simulink model "Platoon_Local_new_2015a"  (R2015a)
settings: Solver=ode45  StartTime=0.0  StopTime=100  RelTol=1e-3
undefined symbols (not defined in the file or in its folder): L, point_character, theta0, V0, x0, z0
undefined symbols (not defined in the file): theta1, theta2, theta3, theta4, x1, x2, x3, x4, z1, z2, z3, z4
settings Model: Creator=Prajval  LastModifiedBy=Aman
settings DataIOCC: LimitDataPoints=off  SaveFormat=Dataset
settings HardwareCC: ProdBitPerPointer=64  ProdLargestAtomicFloat=Float  ProdIntDivRoundTo=Zero  ProdEndianess=LittleEndian  ProdHWDeviceType=Specified
settings ModelReferenceCC: PropagateSignalLabelsOutOfModel=on

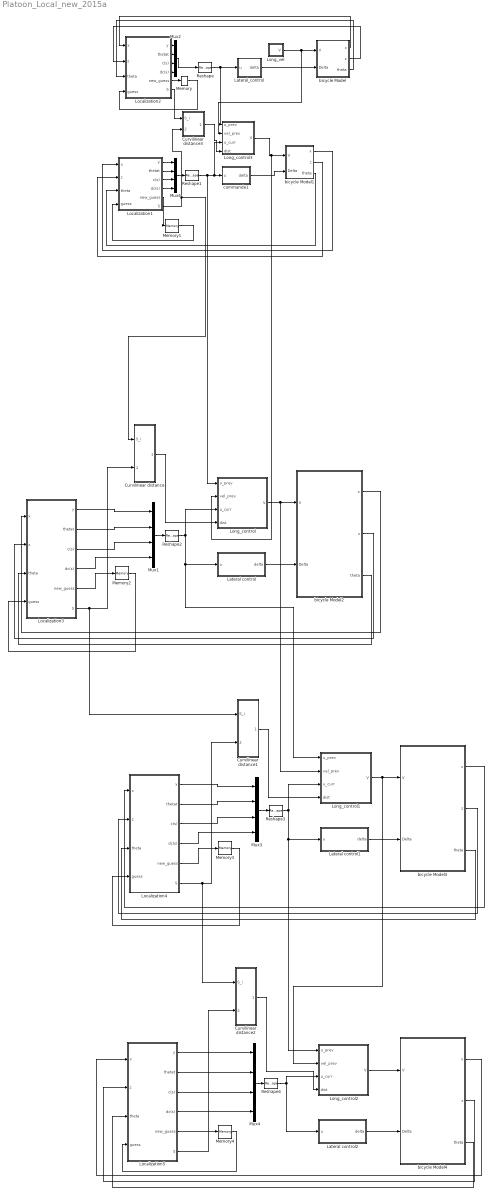
== system Platoon_Local_new_2015a ==
  Curvilinear distance : Subsystem
  Curvilinear distance1 : Subsystem
  Curvilinear distance2 : Subsystem
  Curvilinear distance3 : Subsystem
  Lateral control : MATLAB Function  TreatAsAtomicUnit=on
      settings: PermitHierarchicalResolution=ParametersOnly
  Lateral control1 : MATLAB Function  TreatAsAtomicUnit=on
      settings: PermitHierarchicalResolution=ParametersOnly
  Lateral control2 : MATLAB Function  TreatAsAtomicUnit=on
      settings: PermitHierarchicalResolution=ParametersOnly
  Lateral_control : MATLAB Function  TreatAsAtomicUnit=on
      settings: PermitHierarchicalResolution=ParametersOnly
  Localization1 : Subsystem
  Localization2 : Subsystem
  Localization3 : Subsystem
  Localization4 : Subsystem
  Localization5 : Subsystem
  Long_control : Subsystem
  Long_control1 : Subsystem
  Long_control2 : Subsystem
  Long_control3 : Subsystem
  Long_vel : Subsystem
  Memory{,1..4} (5 alike) : Memory  X0=1
  Mux{1..4,6} (5 alike) : Mux
  Reshape{,1..4} (5 alike) : Reshape  OutputDimensionality=Customize  OutputDimensions=[1,4]
  bicycle Model : Subsystem  mask{L=L, x0=x0, z0=z0, theta0=theta0}
      mask prompts: L "Wheelbase"
  bicycle Model1 : Subsystem  mask{L=L, x0=x1, z0=z1, theta0=theta1}
      mask prompts: L "Wheelbase"
  bicycle Model2 : Subsystem  mask{L=L, x0=x2, z0=z2, theta0=theta2}
      mask prompts: L "Wheelbase"
  bicycle Model3 : Subsystem  mask{L=L, x0=x3, z0=z3, theta0=theta3}
      mask prompts: L "Wheelbase"
  bicycle Model4 : Subsystem  mask{L=L, x0=x4, z0=z4, theta0=theta4}
      mask prompts: L "Wheelbase"
  commande1 : MATLAB Function  TreatAsAtomicUnit=on
      settings: PermitHierarchicalResolution=ParametersOnly
  wires:
  Lateral_control/1(delta) -> bicycle Model/2("Delta ")
  commande1/1(delta) -> bicycle Model1/2("Delta ")
  Mux6/1 -> Reshape1/1
  Localization2/3(c(s)) -> Mux2/3
  Localization2/2(thetat) -> Mux2/2
  Localization2/1(y) -> Mux2/1
  Reshape/1 -> Long_control3/1(u_prev), Lateral_control/1(u)
  Localization2/4(dc(s)) -> Mux2/4
  Mux2/1 -> Reshape/1
  Localization2/5("new_guess ") -> Memory/1
  bicycle Model/1(x) -> Localization2/1(x)
  bicycle Model/2(z) -> Localization2/2(z)
  bicycle Model/3(theta) -> Localization2/3(theta)
  Memory/1 -> Localization2/4(guess)
  Localization1/1(y) -> Mux6/1
  Localization1/2(thetat) -> Mux6/2
  Localization1/3(c(s)) -> Mux6/3
  Localization1/4(dc(s)) -> Mux6/4
  Localization1/5("new_guess ") -> Memory1/1
  Memory1/1 -> Localization1/4(guess)
  Localization1/6(S) -> Curvilinear distance3/2(S_i+1), Curvilinear distance/1(S_i)
  Reshape1/1 -> commande1/1(u), Long_control3/3(u_curr), Long_control/1(u_prev)
  bicycle Model1/1(x) -> Localization1/1(x)
  bicycle Model1/2(z) -> Localization1/2(z)
  bicycle Model1/3(theta) -> Localization1/3(theta)
  Lateral control/1(delta) -> bicycle Model2/2("Delta ")
  Mux1/1 -> Reshape2/1
  Localization3/1(y) -> Mux1/1
  Localization3/2(thetat) -> Mux1/2
  Localization3/3(c(s)) -> Mux1/3
  Localization3/4(dc(s)) -> Mux1/4
  Localization3/5("new_guess ") -> Memory2/1
  Reshape2/1 -> Long_control1/1(u_prev), Lateral control/1(u), Long_control/3(u_curr)
  bicycle Model2/1(x) -> Localization3/1(x)
  bicycle Model2/2(z) -> Localization3/2(z)
  bicycle Model2/3(theta) -> Localization3/3(theta)
  Long_control/1(V) -> Long_control1/2(vel_prev), bicycle Model2/1(V)
  Memory2/1 -> Localization3/4(guess)
  Localization3/6(S) -> Curvilinear distance1/1(S_i), Curvilinear distance/2(S_i+1)
  Curvilinear distance/1(dist) -> Long_control/4(dist)
  Lateral control1/1(delta) -> bicycle Model3/2("Delta ")
  Mux3/1 -> Reshape3/1
  Localization4/1(y) -> Mux3/1
  Localization4/2(thetat) -> Mux3/2
  Localization4/3(c(s)) -> Mux3/3
  Localization4/4(dc(s)) -> Mux3/4
  Localization4/5("new_guess ") -> Memory3/1
  Reshape3/1 -> Long_control2/1(u_prev), Lateral control1/1(u), Long_control1/3(u_curr)
  bicycle Model3/1(x) -> Localization4/1(x)
  bicycle Model3/2(z) -> Localization4/2(z)
  bicycle Model3/3(theta) -> Localization4/3(theta)
  Long_control1/1(V) -> Long_control2/2(vel_prev), bicycle Model3/1(V)
  Memory3/1 -> Localization4/4(guess)
  Curvilinear distance1/1(dist) -> Long_control1/4(dist)
  Lateral control2/1(delta) -> bicycle Model4/2("Delta ")
  Mux4/1 -> Reshape4/1
  Localization5/1(y) -> Mux4/1
  Localization5/2(thetat) -> Mux4/2
  Localization5/3(c(s)) -> Mux4/3
  Localization5/4(dc(s)) -> Mux4/4
  Localization5/5("new_guess ") -> Memory4/1
  Reshape4/1 -> Long_control2/3(u_curr), Lateral control2/1(u)
  bicycle Model4/1(x) -> Localization5/1(x)
  bicycle Model4/2(z) -> Localization5/2(z)
  bicycle Model4/3(theta) -> Localization5/3(theta)
  Long_control2/1(V) -> bicycle Model4/1(V)
  Memory4/1 -> Localization5/4(guess)
  Localization5/6(S) -> Curvilinear distance2/2(S_i+1)
  Curvilinear distance2/1(dist) -> Long_control2/4(dist)
  Localization4/6(S) -> Curvilinear distance2/1(S_i), Curvilinear distance1/2(S_i+1)
  Long_vel/1(V) -> Long_control3/2(vel_prev), bicycle Model/1(V)
  Localization2/6(S) -> Curvilinear distance3/1(S_i)
  Long_control3/1(V) -> Long_control/2(vel_prev), bicycle Model1/1(V)
  Curvilinear distance3/1(dist) -> Long_control3/4(dist)

== system Platoon_Local_new_2015a/Curvilinear distance ==
  S_i : Inport
  S_i+1 : Inport  Port=2
  Interpreted MATLAB Function1 : MATLABFcn  MATLABFcn=curv_dist  OutputDimensions=1
  Mux4 : Mux  Inputs=2
  To Workspace2 : ToWorkspace  VariableName=LongErr2  SaveFormat=Timeseries  SampleTime=-1
  dist : Outport
  wires:
  Interpreted MATLAB Function1/1 -> dist/1, To Workspace2/1
  Mux4/1 -> Interpreted MATLAB Function1/1
  S_i/1 -> Mux4/1
  S_i+1/1 -> Mux4/2

== system Platoon_Local_new_2015a/Curvilinear distance1 ==
  S_i : Inport
  S_i+1 : Inport  Port=2
  Interpreted MATLAB Function1 : MATLABFcn  MATLABFcn=curv_dist  OutputDimensions=1
  Mux4 : Mux  Inputs=2
  To Workspace2 : ToWorkspace  VariableName=LongErr3  SaveFormat=Timeseries  SampleTime=-1
  dist : Outport
  wires:
  Interpreted MATLAB Function1/1 -> dist/1, To Workspace2/1
  Mux4/1 -> Interpreted MATLAB Function1/1
  S_i/1 -> Mux4/1
  S_i+1/1 -> Mux4/2

== system Platoon_Local_new_2015a/Curvilinear distance2 ==
  S_i : Inport
  S_i+1 : Inport  Port=2
  Interpreted MATLAB Function1 : MATLABFcn  MATLABFcn=curv_dist  OutputDimensions=1
  Mux4 : Mux  Inputs=2
  To Workspace2 : ToWorkspace  VariableName=LongErr4  SaveFormat=Timeseries  SampleTime=-1
  dist : Outport
  wires:
  Interpreted MATLAB Function1/1 -> dist/1, To Workspace2/1
  Mux4/1 -> Interpreted MATLAB Function1/1
  S_i/1 -> Mux4/1
  S_i+1/1 -> Mux4/2

== system Platoon_Local_new_2015a/Curvilinear distance3 ==
  S_i : Inport
  S_i+1 : Inport  Port=2
  Interpreted MATLAB Function1 : MATLABFcn  MATLABFcn=curv_dist  OutputDimensions=1
  Mux4 : Mux  Inputs=2
  To Workspace2 : ToWorkspace  VariableName=LongErr1  SaveFormat=Timeseries  SampleTime=-1
  dist : Outport
  wires:
  Interpreted MATLAB Function1/1 -> dist/1, To Workspace2/1
  Mux4/1 -> Interpreted MATLAB Function1/1
  S_i/1 -> Mux4/1
  S_i+1/1 -> Mux4/2

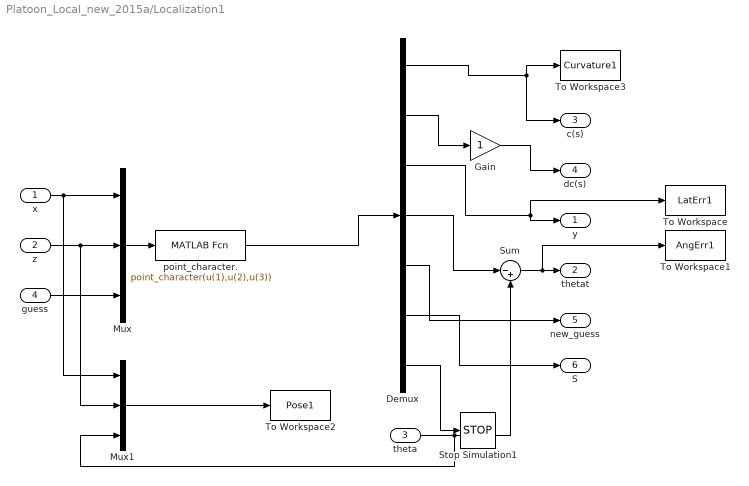
== system Platoon_Local_new_2015a/Localization1 ==
  x : Inport
  z : Inport  Port=2
  theta : Inport  Port=3
  guess : Inport  Port=4
  Demux : Demux  Outputs=7
  Gain : Gain
  Mux : Mux  Inputs=3
  Mux1 : Mux  Inputs=3
  Stop Simulation1 : Stop
  Sum : Sum  Inputs=|-+
  To Workspace : ToWorkspace  VariableName=LatErr1  SaveFormat=Timeseries  SampleTime=-1
  To Workspace1 : ToWorkspace  VariableName=AngErr1  SaveFormat=Timeseries  SampleTime=-1
  To Workspace2 : ToWorkspace  VariableName=Pose1  SaveFormat=Timeseries  SampleTime=-1
  To Workspace3 : ToWorkspace  VariableName=Curvature1  SaveFormat=Timeseries  SampleTime=-1
  point_character. : MATLABFcn  MATLABFcn=point_character(u(1),u(2),u(3))  OutputDimensions=7  OutputSignalType=real  Output1D=off
  y : Outport
  thetat : Outport  Port=2
  c(s) : Outport  Port=3
  dc(s) : Outport  Port=4
  "new_guess " : Outport  Port=5
  S : Outport  Port=6
  wires:
  x/1 -> Mux1/1, Mux/1
  guess/1 -> Mux/3
  z/1 -> Mux1/2, Mux/2
  theta/1 -> Mux1/3, Sum/2
  Mux1/1 -> To Workspace2/1
  Demux/1 -> c(s)/1, To Workspace3/1
  Demux/3 -> y/1, To Workspace/1
  Demux/4 -> Sum/1
  Sum/1 -> To Workspace1/1, thetat/1
  Demux/5 -> "new_guess "/1
  Mux/1 -> point_character./1
  point_character./1 -> Demux/1
  Demux/2 -> Gain/1
  Gain/1 -> dc(s)/1
  Demux/6 -> S/1
  Demux/7 -> Stop Simulation1/1

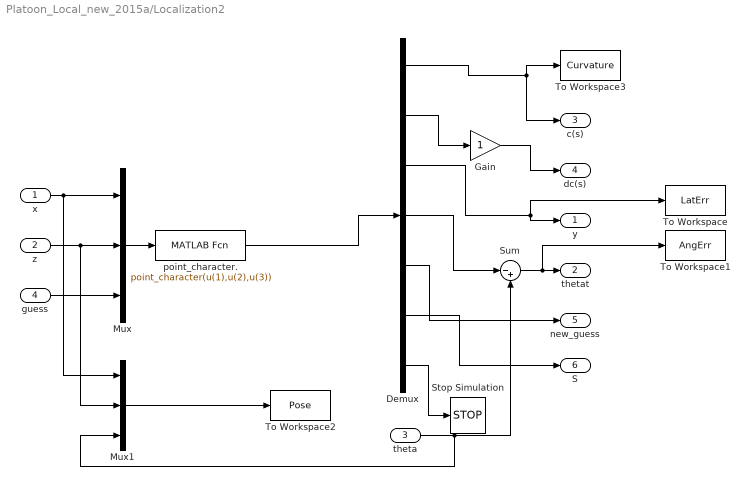
== system Platoon_Local_new_2015a/Localization2 ==
  x : Inport
  z : Inport  Port=2
  theta : Inport  Port=3
  guess : Inport  Port=4
  Demux : Demux  Outputs=7
  Gain : Gain
  Mux : Mux  Inputs=3
  Mux1 : Mux  Inputs=3
  Stop Simulation : Stop
  Sum : Sum  Inputs=|-+
  To Workspace : ToWorkspace  VariableName=LatErr  SaveFormat=Timeseries  SampleTime=-1
  To Workspace1 : ToWorkspace  VariableName=AngErr  SaveFormat=Timeseries  SampleTime=-1
  To Workspace2 : ToWorkspace  VariableName=Pose  SaveFormat=Timeseries  SampleTime=-1
  To Workspace3 : ToWorkspace  VariableName=Curvature  SaveFormat=Timeseries  SampleTime=-1
  point_character. : MATLABFcn  MATLABFcn=point_character(u(1),u(2),u(3))  OutputDimensions=7  OutputSignalType=real  Output1D=off
  y : Outport
  thetat : Outport  Port=2
  c(s) : Outport  Port=3
  dc(s) : Outport  Port=4
  "new_guess " : Outport  Port=5
  S : Outport  Port=6
  wires:
  x/1 -> Mux1/1, Mux/1
  guess/1 -> Mux/3
  z/1 -> Mux1/2, Mux/2
  theta/1 -> Mux1/3, Sum/2
  Mux1/1 -> To Workspace2/1
  Demux/1 -> c(s)/1, To Workspace3/1
  Demux/3 -> y/1, To Workspace/1
  Demux/4 -> Sum/1
  Sum/1 -> To Workspace1/1, thetat/1
  Demux/5 -> "new_guess "/1
  Mux/1 -> point_character./1
  point_character./1 -> Demux/1
  Demux/2 -> Gain/1
  Gain/1 -> dc(s)/1
  Demux/6 -> S/1
  Demux/7 -> Stop Simulation/1

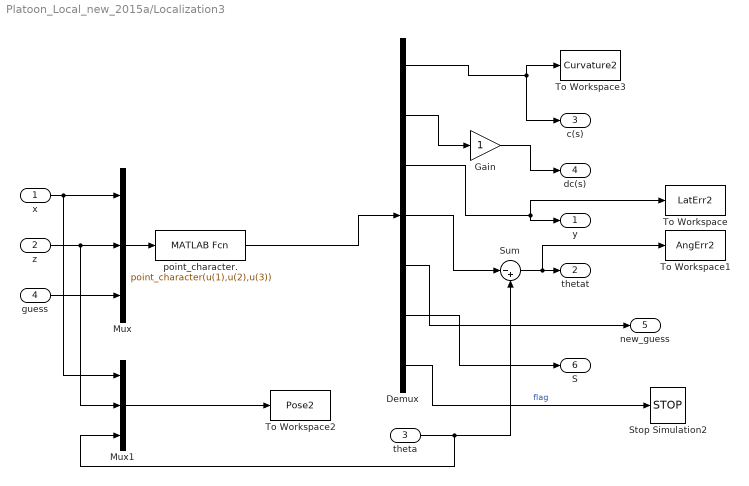
== system Platoon_Local_new_2015a/Localization3 ==
  x : Inport
  z : Inport  Port=2
  theta : Inport  Port=3
  guess : Inport  Port=4
  Demux : Demux  Outputs=7
  Gain : Gain
  Mux : Mux  Inputs=3
  Mux1 : Mux  Inputs=3
  Stop Simulation2 : Stop
  Sum : Sum  Inputs=|-+
  To Workspace : ToWorkspace  VariableName=LatErr2  SaveFormat=Timeseries  SampleTime=-1
  To Workspace1 : ToWorkspace  VariableName=AngErr2  SaveFormat=Timeseries  SampleTime=-1
  To Workspace2 : ToWorkspace  VariableName=Pose2  SaveFormat=Timeseries  SampleTime=-1
  To Workspace3 : ToWorkspace  VariableName=Curvature2  SaveFormat=Timeseries  SampleTime=-1
  point_character. : MATLABFcn  MATLABFcn=point_character(u(1),u(2),u(3))  OutputDimensions=7  OutputSignalType=real  Output1D=off
  y : Outport
  thetat : Outport  Port=2
  c(s) : Outport  Port=3
  dc(s) : Outport  Port=4
  "new_guess " : Outport  Port=5
  S : Outport  Port=6
  wires:
  x/1 -> Mux1/1, Mux/1
  guess/1 -> Mux/3
  z/1 -> Mux1/2, Mux/2
  theta/1 -> Mux1/3, Sum/2
  Mux1/1 -> To Workspace2/1
  Demux/1 -> c(s)/1, To Workspace3/1
  Demux/3 -> y/1, To Workspace/1
  Demux/4 -> Sum/1
  Sum/1 -> To Workspace1/1, thetat/1
  Mux/1 -> point_character./1
  point_character./1 -> Demux/1
  Demux/2 -> Gain/1
  Gain/1 -> dc(s)/1
  Demux/6 -> S/1
  Demux/5 -> "new_guess "/1
  Demux/7 -> Stop Simulation2/1  "flag"

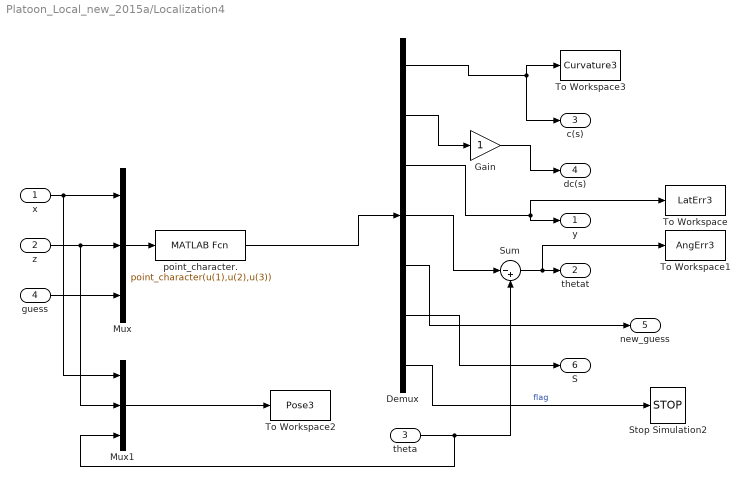
== system Platoon_Local_new_2015a/Localization4 ==
  x : Inport
  z : Inport  Port=2
  theta : Inport  Port=3
  guess : Inport  Port=4
  Demux : Demux  Outputs=7
  Gain : Gain
  Mux : Mux  Inputs=3
  Mux1 : Mux  Inputs=3
  Stop Simulation2 : Stop
  Sum : Sum  Inputs=|-+
  To Workspace : ToWorkspace  VariableName=LatErr3  SaveFormat=Timeseries  SampleTime=-1
  To Workspace1 : ToWorkspace  VariableName=AngErr3  SaveFormat=Timeseries  SampleTime=-1
  To Workspace2 : ToWorkspace  VariableName=Pose3  SaveFormat=Timeseries  SampleTime=-1
  To Workspace3 : ToWorkspace  VariableName=Curvature3  SaveFormat=Timeseries  SampleTime=-1
  point_character. : MATLABFcn  MATLABFcn=point_character(u(1),u(2),u(3))  OutputDimensions=7  OutputSignalType=real  Output1D=off
  y : Outport
  thetat : Outport  Port=2
  c(s) : Outport  Port=3
  dc(s) : Outport  Port=4
  "new_guess " : Outport  Port=5
  S : Outport  Port=6
  wires:
  x/1 -> Mux1/1, Mux/1
  guess/1 -> Mux/3
  z/1 -> Mux1/2, Mux/2
  theta/1 -> Mux1/3, Sum/2
  Mux1/1 -> To Workspace2/1
  Demux/1 -> c(s)/1, To Workspace3/1
  Demux/3 -> y/1, To Workspace/1
  Demux/4 -> Sum/1
  Sum/1 -> To Workspace1/1, thetat/1
  Mux/1 -> point_character./1
  point_character./1 -> Demux/1
  Demux/2 -> Gain/1
  Gain/1 -> dc(s)/1
  Demux/6 -> S/1
  Demux/5 -> "new_guess "/1
  Demux/7 -> Stop Simulation2/1  "flag"

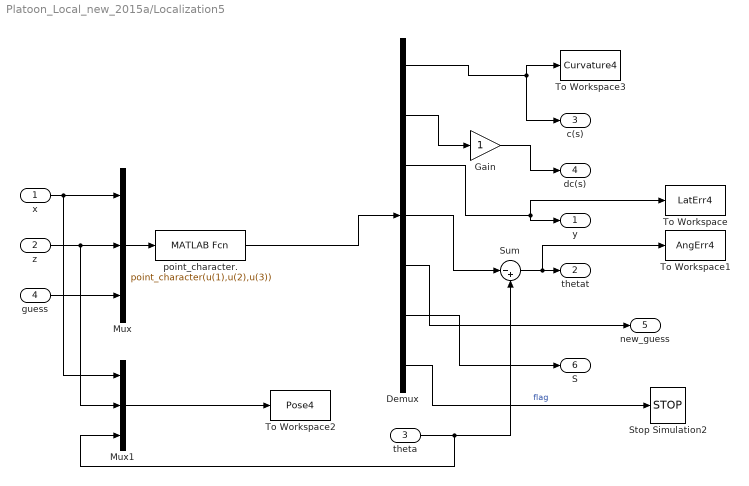
== system Platoon_Local_new_2015a/Localization5 ==
  x : Inport
  z : Inport  Port=2
  theta : Inport  Port=3
  guess : Inport  Port=4
  Demux : Demux  Outputs=7
  Gain : Gain
  Mux : Mux  Inputs=3
  Mux1 : Mux  Inputs=3
  Stop Simulation2 : Stop
  Sum : Sum  Inputs=|-+
  To Workspace : ToWorkspace  VariableName=LatErr4  SaveFormat=Timeseries  SampleTime=-1
  To Workspace1 : ToWorkspace  VariableName=AngErr4  SaveFormat=Timeseries  SampleTime=-1
  To Workspace2 : ToWorkspace  VariableName=Pose4  SaveFormat=Timeseries  SampleTime=-1
  To Workspace3 : ToWorkspace  VariableName=Curvature4  SaveFormat=Timeseries  SampleTime=-1
  point_character. : MATLABFcn  MATLABFcn=point_character(u(1),u(2),u(3))  OutputDimensions=7  OutputSignalType=real  Output1D=off
  y : Outport
  thetat : Outport  Port=2
  c(s) : Outport  Port=3
  dc(s) : Outport  Port=4
  "new_guess " : Outport  Port=5
  S : Outport  Port=6
  wires:
  x/1 -> Mux1/1, Mux/1
  guess/1 -> Mux/3
  z/1 -> Mux1/2, Mux/2
  theta/1 -> Mux1/3, Sum/2
  Mux1/1 -> To Workspace2/1
  Demux/1 -> c(s)/1, To Workspace3/1
  Demux/3 -> y/1, To Workspace/1
  Demux/4 -> Sum/1
  Sum/1 -> To Workspace1/1, thetat/1
  Mux/1 -> point_character./1
  point_character./1 -> Demux/1
  Demux/2 -> Gain/1
  Gain/1 -> dc(s)/1
  Demux/6 -> S/1
  Demux/5 -> "new_guess "/1
  Demux/7 -> Stop Simulation2/1  "flag"

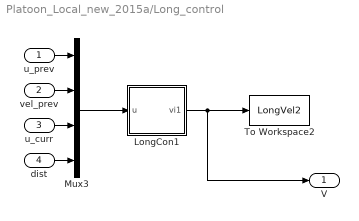
== system Platoon_Local_new_2015a/Long_control ==
  u_prev : Inport
  vel_prev : Inport  Port=2
  u_curr : Inport  Port=3
  dist : Inport  Port=4
  LongCon1 : MATLAB Function  TreatAsAtomicUnit=on
      settings: PermitHierarchicalResolution=ParametersOnly
  Mux3 : Mux
  To Workspace2 : ToWorkspace  VariableName=LongVel2  SaveFormat=Timeseries  SampleTime=-1
  V : Outport
  wires:
  LongCon1/1(vi1) -> V/1, To Workspace2/1
  Mux3/1 -> LongCon1/1(u)
  u_prev/1 -> Mux3/1
  u_curr/1 -> Mux3/3
  dist/1 -> Mux3/4
  vel_prev/1 -> Mux3/2

== system Platoon_Local_new_2015a/Long_control1 ==
  u_prev : Inport
  vel_prev : Inport  Port=2
  u_curr : Inport  Port=3
  dist : Inport  Port=4
  LongCon1 : MATLAB Function  TreatAsAtomicUnit=on
      settings: PermitHierarchicalResolution=ParametersOnly
  Mux3 : Mux
  To Workspace2 : ToWorkspace  VariableName=LongVel3  SaveFormat=Timeseries  SampleTime=-1
  V : Outport
  wires:
  LongCon1/1(vi1) -> V/1, To Workspace2/1
  Mux3/1 -> LongCon1/1(u)
  u_prev/1 -> Mux3/1
  u_curr/1 -> Mux3/3
  dist/1 -> Mux3/4
  vel_prev/1 -> Mux3/2

== system Platoon_Local_new_2015a/Long_control2 ==
  u_prev : Inport
  vel_prev : Inport  Port=2
  u_curr : Inport  Port=3
  dist : Inport  Port=4
  LongCon1 : MATLAB Function  TreatAsAtomicUnit=on
      settings: PermitHierarchicalResolution=ParametersOnly
  Mux3 : Mux
  To Workspace2 : ToWorkspace  VariableName=LongVel4  SaveFormat=Timeseries  SampleTime=-1
  V : Outport
  wires:
  LongCon1/1(vi1) -> V/1, To Workspace2/1
  Mux3/1 -> LongCon1/1(u)
  u_prev/1 -> Mux3/1
  u_curr/1 -> Mux3/3
  dist/1 -> Mux3/4
  vel_prev/1 -> Mux3/2

== system Platoon_Local_new_2015a/Long_control3 ==
  u_prev : Inport
  vel_prev : Inport  Port=2
  u_curr : Inport  Port=3
  dist : Inport  Port=4
  LongCon1 : MATLAB Function  TreatAsAtomicUnit=on
      settings: PermitHierarchicalResolution=ParametersOnly
  Mux3 : Mux
  To Workspace2 : ToWorkspace  VariableName=LongVel1  SaveFormat=Timeseries  SampleTime=-1
  V : Outport
  wires:
  LongCon1/1(vi1) -> V/1, To Workspace2/1
  Mux3/1 -> LongCon1/1(u)
  u_prev/1 -> Mux3/1
  u_curr/1 -> Mux3/3
  dist/1 -> Mux3/4
  vel_prev/1 -> Mux3/2

== system Platoon_Local_new_2015a/Long_vel ==
  Longiitudinal Velocity : Constant  Value=V0
  To Workspace5 : ToWorkspace  VariableName=LongVel  SaveFormat=Timeseries  SampleTime=-1
  V : Outport
  wires:
  Longiitudinal Velocity/1 -> V/1, To Workspace5/1

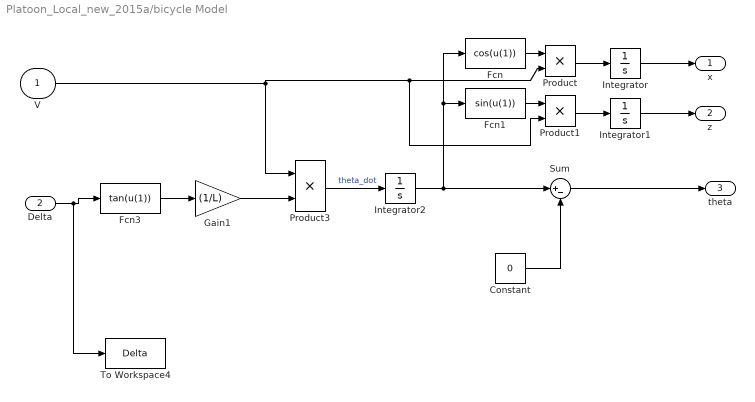
== system Platoon_Local_new_2015a/bicycle Model ==
  V : Inport
  "Delta " : Inport  Port=2
  Constant : Constant  Value=0
  Fcn : Fcn  Expr=cos(u(1))
  Fcn1 : Fcn  Expr=sin(u(1))
  Fcn3 : Fcn  Expr=tan(u(1))
  Gain1 : Gain  Gain=(1/L)
  Integrator : Integrator  InitialCondition=x0
  Integrator1 : Integrator  InitialCondition=z0
  Integrator2 : Integrator  InitialCondition=theta0
  Product : Product
  Product1 : Product
  Product3 : Product
  Sum : Sum  Inputs=|+-
  To Workspace4 : ToWorkspace  VariableName=Delta  SaveFormat=Timeseries  SampleTime=-1
  x : Outport
  z : Outport  Port=2
  theta : Outport  Port=3
  wires:
  Integrator/1 -> x/1
  Integrator2/1 -> Sum/1, Fcn1/1, Fcn/1
  Integrator1/1 -> z/1
  Fcn/1 -> Product/1
  Product1/1 -> Integrator1/1
  Gain1/1 -> Product3/2
  Fcn1/1 -> Product1/1
  V/1 -> Product3/1, Product1/2, Product/2
  Product/1 -> Integrator/1
  Fcn3/1 -> Gain1/1
  Product3/1 -> Integrator2/1  "theta_dot"
  Constant/1 -> Sum/2
  Sum/1 -> theta/1
  "Delta "/1 -> To Workspace4/1, Fcn3/1

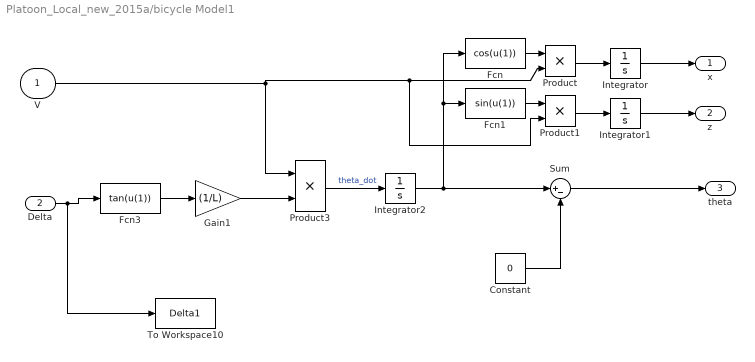
== system Platoon_Local_new_2015a/bicycle Model1 ==
  V : Inport
  "Delta " : Inport  Port=2
  Constant : Constant  Value=0
  Fcn : Fcn  Expr=cos(u(1))
  Fcn1 : Fcn  Expr=sin(u(1))
  Fcn3 : Fcn  Expr=tan(u(1))
  Gain1 : Gain  Gain=(1/L)
  Integrator : Integrator  InitialCondition=x0
  Integrator1 : Integrator  InitialCondition=z0
  Integrator2 : Integrator  InitialCondition=theta0
  Product : Product
  Product1 : Product
  Product3 : Product
  Sum : Sum  Inputs=|+-
  To Workspace10 : ToWorkspace  VariableName=Delta1  SaveFormat=Timeseries  SampleTime=-1
  x : Outport
  z : Outport  Port=2
  theta : Outport  Port=3
  wires:
  Integrator/1 -> x/1
  Integrator2/1 -> Sum/1, Fcn1/1, Fcn/1
  Integrator1/1 -> z/1
  Fcn/1 -> Product/1
  Product1/1 -> Integrator1/1
  Gain1/1 -> Product3/2
  Fcn1/1 -> Product1/1
  V/1 -> Product3/1, Product1/2, Product/2
  Product/1 -> Integrator/1
  Fcn3/1 -> Gain1/1
  "Delta "/1 -> To Workspace10/1, Fcn3/1
  Product3/1 -> Integrator2/1  "theta_dot"
  Constant/1 -> Sum/2
  Sum/1 -> theta/1

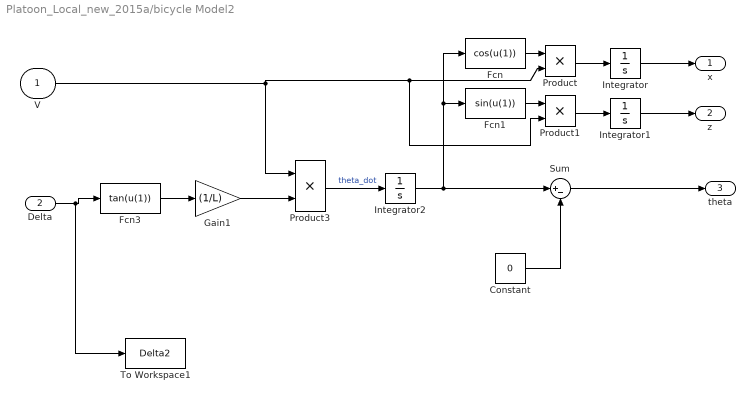
== system Platoon_Local_new_2015a/bicycle Model2 ==
  V : Inport
  "Delta " : Inport  Port=2
  Constant : Constant  Value=0
  Fcn : Fcn  Expr=cos(u(1))
  Fcn1 : Fcn  Expr=sin(u(1))
  Fcn3 : Fcn  Expr=tan(u(1))
  Gain1 : Gain  Gain=(1/L)
  Integrator : Integrator  InitialCondition=x0
  Integrator1 : Integrator  InitialCondition=z0
  Integrator2 : Integrator  InitialCondition=theta0
  Product : Product
  Product1 : Product
  Product3 : Product
  Sum : Sum  Inputs=|+-
  To Workspace1 : ToWorkspace  VariableName=Delta2  SaveFormat=Timeseries  SampleTime=-1
  x : Outport
  z : Outport  Port=2
  theta : Outport  Port=3
  wires:
  Integrator/1 -> x/1
  Integrator2/1 -> Sum/1, Fcn1/1, Fcn/1
  Integrator1/1 -> z/1
  Fcn/1 -> Product/1
  Product1/1 -> Integrator1/1
  Gain1/1 -> Product3/2
  Fcn1/1 -> Product1/1
  V/1 -> Product3/1, Product1/2, Product/2
  Product/1 -> Integrator/1
  Fcn3/1 -> Gain1/1
  Product3/1 -> Integrator2/1  "theta_dot"
  Constant/1 -> Sum/2
  Sum/1 -> theta/1
  "Delta "/1 -> To Workspace1/1, Fcn3/1

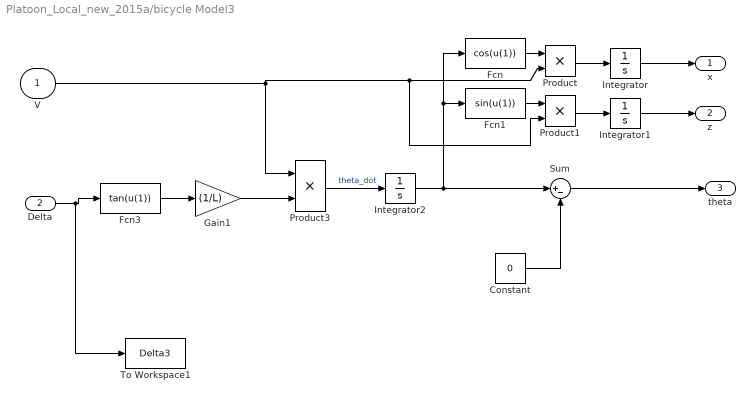
== system Platoon_Local_new_2015a/bicycle Model3 ==
  V : Inport
  "Delta " : Inport  Port=2
  Constant : Constant  Value=0
  Fcn : Fcn  Expr=cos(u(1))
  Fcn1 : Fcn  Expr=sin(u(1))
  Fcn3 : Fcn  Expr=tan(u(1))
  Gain1 : Gain  Gain=(1/L)
  Integrator : Integrator  InitialCondition=x0
  Integrator1 : Integrator  InitialCondition=z0
  Integrator2 : Integrator  InitialCondition=theta0
  Product : Product
  Product1 : Product
  Product3 : Product
  Sum : Sum  Inputs=|+-
  To Workspace1 : ToWorkspace  VariableName=Delta3  SaveFormat=Timeseries  SampleTime=-1
  x : Outport
  z : Outport  Port=2
  theta : Outport  Port=3
  wires:
  Integrator/1 -> x/1
  Integrator2/1 -> Sum/1, Fcn1/1, Fcn/1
  Integrator1/1 -> z/1
  Fcn/1 -> Product/1
  Product1/1 -> Integrator1/1
  Gain1/1 -> Product3/2
  Fcn1/1 -> Product1/1
  V/1 -> Product3/1, Product1/2, Product/2
  Product/1 -> Integrator/1
  Fcn3/1 -> Gain1/1
  Product3/1 -> Integrator2/1  "theta_dot"
  Constant/1 -> Sum/2
  Sum/1 -> theta/1
  "Delta "/1 -> To Workspace1/1, Fcn3/1

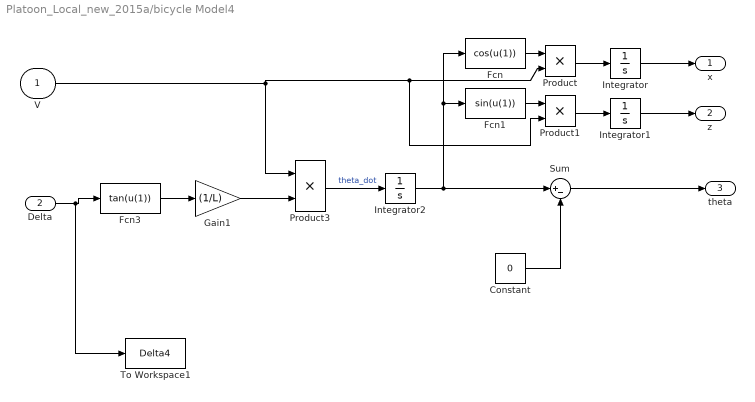
== system Platoon_Local_new_2015a/bicycle Model4 ==
  V : Inport
  "Delta " : Inport  Port=2
  Constant : Constant  Value=0
  Fcn : Fcn  Expr=cos(u(1))
  Fcn1 : Fcn  Expr=sin(u(1))
  Fcn3 : Fcn  Expr=tan(u(1))
  Gain1 : Gain  Gain=(1/L)
  Integrator : Integrator  InitialCondition=x0
  Integrator1 : Integrator  InitialCondition=z0
  Integrator2 : Integrator  InitialCondition=theta0
  Product : Product
  Product1 : Product
  Product3 : Product
  Sum : Sum  Inputs=|+-
  To Workspace1 : ToWorkspace  VariableName=Delta4  SaveFormat=Timeseries  SampleTime=-1
  x : Outport
  z : Outport  Port=2
  theta : Outport  Port=3
  wires:
  Integrator/1 -> x/1
  Integrator2/1 -> Sum/1, Fcn1/1, Fcn/1
  Integrator1/1 -> z/1
  Fcn/1 -> Product/1
  Product1/1 -> Integrator1/1
  Gain1/1 -> Product3/2
  Fcn1/1 -> Product1/1
  V/1 -> Product3/1, Product1/2, Product/2
  Product/1 -> Integrator/1
  Fcn3/1 -> Gain1/1
  Product3/1 -> Integrator2/1  "theta_dot"
  Constant/1 -> Sum/2
  Sum/1 -> theta/1
  "Delta "/1 -> To Workspace1/1, Fcn3/1

== matlab function Platoon_Local_new_2015a/Lateral control ==
  data: u input; delta output
function delta  = fcn(u)
Kd=10; % Robotic Trajectory 
Kp=25;

%Kd = 1; % Traj Z Adams Trajectory.
%Kp = 0.25;

%Kd = 2; % Line
%Kp = 1;

%Kd = 1;
%Kp = 2;

L=1;
yi=u(1);
tetati=u(2);
csi=u(3);
dcsi=u(4);
a=1-csi*yi;
ctetati=cos(tetati);


x=ctetati^3/a^2*(  (dcsi*yi - Kd*a)*tan(tetati)-Kp*yi + csi*a*tan(tetati)^2) + ctetati*csi/a;

delta=atan(L*x);

== matlab function Platoon_Local_new_2015a/Lateral_control ==
  data: u input; delta output
function delta  = fcn(u)
Kd=10; % Robotic Trajectory 
Kp=25;

%Kd = 1; % Traj Z Adams Trajectory.
%Kp = 0.25;

%Kd = 2; % Line
%Kp = 1;

%Kd = 1;
%Kp = 2;

L=1;
yi=u(1);
tetati=u(2);
csi=u(3);
dcsi=u(4);
a=1-csi*yi;
ctetati=cos(tetati);


x=ctetati^3/a^2*(  (dcsi*yi - Kd*a)*tan(tetati)-Kp*yi + csi*a*tan(tetati)^2) + ctetati*csi/a;

delta=atan(L*x);

== matlab function Platoon_Local_new_2015a/commande1 ==
  data: u input; delta output
function delta  = fcn(u)
Kd=10; % Robotic Trajectory 
Kp=25;

%Kd = 1; % Traj Z Adams Trajectory.
%Kp = 0.25;

%Kd = 2; % Line
%Kp = 1;

%Kd = 1;
%Kp = 2;

L=1;
yi=u(1);
tetati=u(2);
csi=u(3);
dcsi=u(4);
a=1-csi*yi;
ctetati=cos(tetati);


x=ctetati^3/a^2*(  (dcsi*yi - Kd*a)*tan(tetati)-Kp*yi + csi*a*tan(tetati)^2) + ctetati*csi/a;

delta=atan(L*x);

== matlab function Platoon_Local_new_2015a/Long_control/LongCon1 ==
  data: u input; vi1 output
function vi1  = fcn(u)
vi1=0;
yi=u(1);
tetati=u(2);
csi=u(3);
dcsi=u(4);
vi=u(5);
yi1=u(6);
tetati1=u(7);
csi1=u(8);
dcsi1=u(9);

a=1-csi*yi;
a1=1-csi1*yi1;
ctetati=cos(tetati);
ctetati1=cos(tetati1);
L=1;
K=5;
d=1;
ei=u(10)-d;


vi1=a1/ctetati1*(vi*ctetati/a + K*ei);

== matlab function Platoon_Local_new_2015a/Long_control3/LongCon1 ==
  data: u input; vi1 output
function vi1  = fcn(u)
vi1=0;
yi=u(1);
tetati=u(2);
csi=u(3);
dcsi=u(4);
vi=u(5);
yi1=u(6);
tetati1=u(7);
csi1=u(8);
dcsi1=u(9);

a=1-csi*yi;
a1=1-csi1*yi1;
ctetati=cos(tetati);
ctetati1=cos(tetati1);
L=1;
K=5;
d=1;
ei=u(10)-d;


vi1=a1/ctetati1*(vi*ctetati/a + K*ei);

== matlab function Platoon_Local_new_2015a/Lateral control1 ==
  data: u input; delta output
function delta  = fcn(u)
Kd=10; % Robotic Trajectory 
Kp=25;

%Kd = 1; % Traj Z Adams Trajectory.
%Kp = 0.25;

%Kd = 2; % Line
%Kp = 1;

%Kd = 1;
%Kp = 2;

L=1;
yi=u(1);
tetati=u(2);
csi=u(3);
dcsi=u(4);
a=1-csi*yi;
ctetati=cos(tetati);


x=ctetati^3/a^2*(  (dcsi*yi - Kd*a)*tan(tetati)-Kp*yi + csi*a*tan(tetati)^2) + ctetati*csi/a;

delta=atan(L*x);

== matlab function Platoon_Local_new_2015a/Long_control1/LongCon1 ==
  data: u input; vi1 output
function vi1  = fcn(u)
vi1=0;
yi=u(1);
tetati=u(2);
csi=u(3);
dcsi=u(4);
vi=u(5);
yi1=u(6);
tetati1=u(7);
csi1=u(8);
dcsi1=u(9);

a=1-csi*yi;
a1=1-csi1*yi1;
ctetati=cos(tetati);
ctetati1=cos(tetati1);
L=1;
K=5;
d=1;
ei=u(10)-d;


vi1=a1/ctetati1*(vi*ctetati/a + K*ei);

== matlab function Platoon_Local_new_2015a/Lateral control2 ==
  data: u input; delta output
function delta  = fcn(u)
Kd=10; % Robotic Trajectory 
Kp=25;

%Kd = 1; % Traj Z Adams Trajectory.
%Kp = 0.25;

%Kd = 2; % Line
%Kp = 1;

%Kd = 1;
%Kp = 2;

L=1;
yi=u(1);
tetati=u(2);
csi=u(3);
dcsi=u(4);
a=1-csi*yi;
ctetati=cos(tetati);


x=ctetati^3/a^2*(  (dcsi*yi - Kd*a)*tan(tetati)-Kp*yi + csi*a*tan(tetati)^2) + ctetati*csi/a;

delta=atan(L*x);

== matlab function Platoon_Local_new_2015a/Long_control2/LongCon1 ==
  data: u input; vi1 output
function vi1  = fcn(u)
vi1=0;
yi=u(1);
tetati=u(2);
csi=u(3);
dcsi=u(4);
vi=u(5);
yi1=u(6);
tetati1=u(7);
csi1=u(8);
dcsi1=u(9);

a=1-csi*yi;
a1=1-csi1*yi1;
ctetati=cos(tetati);
ctetati1=cos(tetati1);
L=1;
K=5;
d=1;
ei=u(10)-d;


vi1=a1/ctetati1*(vi*ctetati/a + K*ei);
